simulink model "AutonomousModel_V1"  (R2020b)
settings: Solver=ode23t  StartTime=0.0  StopTime=180.1  FixedStep=0.05  RelTol=1e-3  EnableMultiTasking=on
model workspace (MAT data in the model file):
  occGrid = robotics.BinaryOccupancyGrid
  occGrid.Grid = [1 1 1 1 1 1 1 1 1 1 1 1 ... (4194304 elements, 2048x2048)]
  occGrid.LayerName = "binaryLayer"
  occGrid.Index = matlabshared.autonomous.internal.CircularBufferIndex
  occGrid.Index.Head = [1 1]
  occGrid.Index.Size = [2048 2048]
  occGrid.Index.NewRegions = [0 0 0 0]
  occGrid.Index.DropEntireMap = 0
  occGrid.Index.DropTwoRegions = [0 0]
  occGrid.Buffer = matlabshared.autonomous.internal.CircularBuffer
  occGrid.Buffer.ConstVal = 0
  occGrid.Buffer.DataType = 'logical'
  occGrid.Buffer.Index = matlabshared.autonomous.internal.CircularBufferIndex
  occGrid.Buffer.Index.Head = [1 1]
  occGrid.Buffer.Index.Size = [2048 2048]
  occGrid.Buffer.Index.NewRegions = [0 0 0 0]
  occGrid.Buffer.Index.DropEntireMap = 0
  occGrid.Buffer.Index.DropTwoRegions = [0 0]
  occGrid.Buffer.Buffer = [1 1 1 1 1 1 1 1 1 1 1 1 ... (4194304 elements, 2048x2048)]
  occGrid.DefaultValueInternal = 0
  occGrid.HasParent = 0
  occGrid.Resolution = 409.6
  occGrid.GridSize = [2048 2048]
  occGrid.GridOriginInLocal = [0 0]
  occGrid.LocalOriginInWorld = [0 0]
  occGrid.Width = 5
  occGrid.Height = 5
  occGrid.LocalOriginInWorldInternal = [0 0]
undefined symbols (not defined in the file): cellLevel, cellPose, cellTypeArray, FloorSurface, isoPoses, platformPoses, PlowSurface, Ref, RobotSurface, WallSurface, X, Y, Z
libraries: sm_lib x286, nesl_utility x157, simulink x72, simulink_extras x2, pid_lib x2
(part 1 of 14)
settings Model: DataTypeOverride=Off  MinMaxOverflowLogging=ForceOff  EnablePacing=on  PacingRate=1000  ExtModeTrigDuration=25  OrderedModelArguments=off  Creator=scastro  LastModifiedBy=wanga
settings SolverCC: AlgebraicLoopSolver=LineSearch
settings DataIOCC: LimitDataPoints=on  SignalLogging=off  ReturnWorkspaceOutputs=off
settings OptimizationCC: DefaultParameterBehavior=Inlined  PassReuseOutputArgsAs=Individual arguments  MaxStackSize=64  EfficientTunableParamExpr=on
settings DebuggingCC: ReadBeforeWriteMsg=DisableAll  WriteAfterWriteMsg=DisableAll  WriteAfterReadMsg=DisableAll  MultiTaskDSMMsg=none  ParameterPrecisionLossMsg=none  ParameterTunabilityLossMsg=error  UnconnectedLineMsg=none  AllowSymbolicDim=off  SFUnexpectedBacktrackingDiag=warning  SFNoUnconditionalDefaultTransitionDiag=warning  SFExecutionAtInitializationDiag=none  ArithmeticOperatorsInVariantConditions=warning
settings HardwareCC: ProdBitPerPointer=32  ProdBitPerSizeT=32  ProdBitPerPtrDiffT=32  ProdLargestAtomicInteger=Long  ProdLargestAtomicFloat=Double  ProdWordSize=32  ProdHWDeviceType=ARM Compatible->ARM Cortex
settings ModelReferenceCC: UpdateModelReferenceTargets=IfOutOfDate
settings SFSimCC: SFSimEcho=off  SimUseLocalCustomCode=off  MATLABDynamicMemAlloc=off  CustomCodeUndefinedFunction=UseInterfaceOnly
settings RTWCC: Description=Embedded Coder  SystemTargetFile=ert.tlc  TemplateMakefile=ert_default_tmf  GenerateReport=on  RTWUseLocalCustomCode=off  Toolchain=GNU Tools for ARM Embedded Processors  IncludeHyperlinkInReport=on  LaunchReport=on  GenerateTraceInfo=on  GenerateTraceReport=on  GenerateTraceReportSl=on  GenerateTraceReportSf=on  GenerateTraceReportEml=on
settings CodeAppCC: ForceParamTrailComments=on  IgnoreCustomStorageClasses=off  OperatorAnnotations=on  SimulinkDataObjDesc=on  SFDataObjDesc=on  InsertBlockDesc=on
settings ERTTargetCC: ExtModeStaticAllocSize=2048  ERTCustomFileTemplate=example_file_process.tlc
settings ConfigComp: CovMetricSettings=dw  CovSaveCumulativeToWorkspaceVar=on  CovSaveSingleToWorkspaceVar=on  CovExternalEMLEnable=off  CovSFcnEnable=off
settings SimscapeCC: SimscapeNominalValues="[{\"value\":\"10\",\"unit\":\"V\"},{\"value\":\"1\",\"unit\":\"A\"},{\"value\":\"10\",\"unit\":\"N*m\"},{\"value\":\"10\",\"unit\":\"bar\"},{\"value\":\"100\",\"unit\":\"kJ/kg\"},{\"value\":\"1\",\"unit\":\"kW\"},{\"value\":\"300\",\"unit\":\"K\"},{\"value\":\"100\",\"unit\":\"cm^3/s\"},{\"value\":\"1\",\"unit\":\"kN\"},{\"value\":\"1\",\"unit\":\"g/cm^3\"},{\"value\":\"1\",\"unit\":\"l\"},{\"value\":\"1\",\"unit\":\"cm^2\"},{\"value\":\"60\",\"unit\":\"Hz\"}]"  SimscapeLogOpenViewer=on  SimscapeLogDataHistory=10000
settings ConfigurationSet: Description=SimMechanics 2G
settings DiagnosticsConfigSet: SimMechanicsRigidlyBoundBlock=none
settings ExplorerConfigSet: InternalSimMechanicsExplorerSettings="<ExplorerConfiguration><canonicalview>default</canonicalview><AnimationSetting><BasePlaybackSpeed>1.0</BasePlaybackSpeed><PlaybackSpeedFactor>1.0</PlaybackSpeedFactor></AnimationSetting><TilePanel><TileInfo><Tiles Columns=\"2\" Count=\"3\" Rows=\"2\"><Column Weight=\"0.5\"/><Column Weight=\"0.5\"/><Row Weight=\"0.6225\"/><Row Weight=\"0.3775\"/><Tile Height=\"1\" Width=\"2\" X=\"0\" Y=\"0\"/><Tile Height=\"1\" Width=\"1\" X=\"0\" Y=\"1\"/><Tile Height=\"1\" Width=\"1\" X=\"1\" Y=\"1\"/></Tiles></TileInfo><SceneInfo><SceneViewer><BGColor><R>0.60000002384185791</R><G>0.60000002384185791</G><B>0.60000002384185791</B></BGColor><Camera><DoPerspective>on</DoPerspective><Position><X>-2.5</X><Y>0</Y><Z>0.469999999999999973</Z></Position><Center><X>-1.56030737921409157</X><Y>0</Y><Z>0.12797985667433126</Z></Center><Up><X>0.342020143325668713</X><Y>0</Y><Z>0.939692620785908428</Z></Up><ViewLimDist>1</ViewLimDist><YLim>0.466307658154998583</YLim><XLim>1.13267634384101279</XLim></Camera></SceneViewer><SceneViewer><BGColor><R>0.60000002384185791</R><G>0.60000002384185791</G><B>0.60000002384185791</B></BGColor><Camera><DoPerspective>off</DoPerspective><Position><X>3.5332314785771386</X><Y>-3.3947402734829315</Y><Z>3.53231830664862745</Z></Position><Center><X>0.446325858412655041</X><Y>-0.728979182990680097</Y><Z>0.58226398573312621</Z></Center><Up><X>-0.344859316417843731</X><Y>0.487999196814355329</Y><Z>0.801828432888458731</Z></Up><ViewLimDist>1</ViewLimDist><YLim>1.33865160703358899</YLim><XLim>2.67730321406717797</XLim></Camera></SceneViewer><SceneViewer><BGColor><R>0.60000002384185791</R><G>0.60000002384185791</G><B>0.60000002384185791</B></BGColor><Camera><DoPerspective>off</DoPerspective><Position><X>-0.106931959652509123</X><Y>-0.225697807623169988</Y><Z>4.9870492424192383</Z></Position><Center><X>-0.106931959652509123</X><Y>-0.225697807623169988</Y><Z>0.219820364094227116</Z></Center><Up><X>0</X><Y>1</Y><Z>-0</Z></Up><ViewLimDist>1</ViewLimDist><YLim>1.8966863569500001</YLim><XLim>3.79337271390000019</XLim></Camera></SceneViewer></SceneInfo></TilePanel><MechEditorPanel><Cameras><Camera><Id>Camera1</Id><Value><Name>RobotView</Name><NativeCamera><PositionTrackingFeature>BEST_Robotics_2020_Game_Double_Click.BEST_2020_Robot.Body.RobotCamera.F</PositionTrackingFeature><CenterTrackingFeature>BEST_Robotics_2020_Game_Double_Click.BEST_2020_Robot.Body.RobotCamera.F</CenterTrackingFeature><UpVectorTrackingFeature>BEST_Robotics_2020_Game_Double_Click.BEST_2020_Robot.Body.RobotCamera.F</UpVectorTrackingFeature><CenterTrackingOrigin>off</CenterTrackingOrigin><CenterTrackingDirection>+X</CenterTrackingDirection><UpVectorTrackingDirection>+Z</UpVectorTrackingDirection></NativeCamera></Value></Camera></Cameras><GfxPanelCameraMap><MapElement CameraMLId=\"Camera1\" GfxPanelIndex=\"0\"/></GfxPanelCameraMap><VideoCreator><PlaybackSpeedRatio>1.0</PlaybackSpeedRatio><FrameRate>16</FrameRate><VideoFormat>Motion JPEG AVI</VideoFormat><FrameSize>auto</FrameSize></VideoCreator></MechEditorPanel></ExplorerConfiguration>"

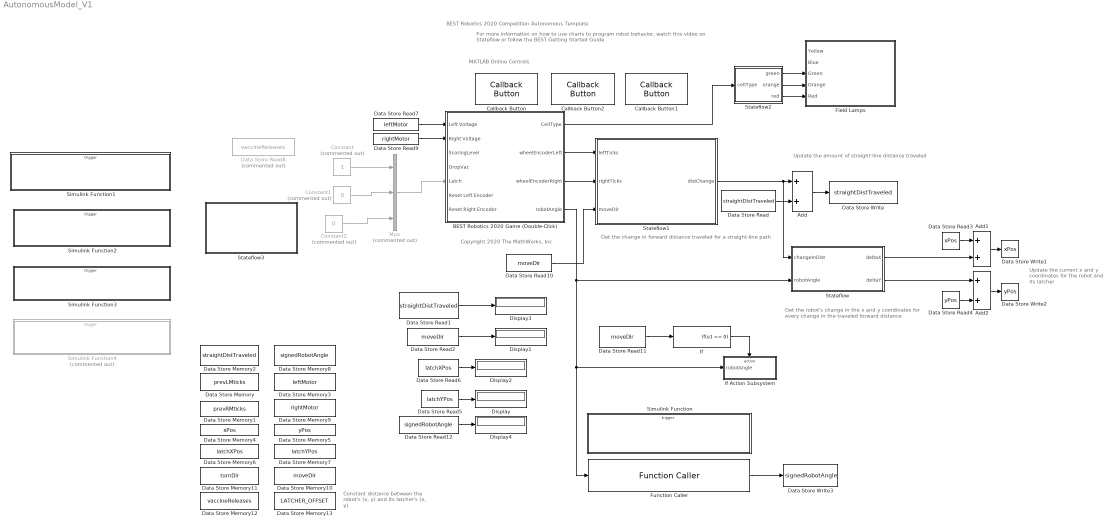
== system AutonomousModel_V1 ==
  note: Update the current x and y coordinates for the robot and its latcher
  note: Get the robot's change in the x and y coordinates for
      | every change in the traveled forward distance
  note: Update the amount of straight-line distance traveled
  note: Get the change in forward distance traveled for a straight-line path
  note: MATLAB Online Controls
  note: For more information on how to use charts to program robot behavior,
      | watch this video on Stateflow or follow the BEST Getting Started Guide
  note: BEST Robotics 2020 Competition Autonomous Template
  note: Copyright 2020 The MathWorks, Inc
  note: Constant distance between the robot's (x, y) and
      | its latcher's (x, y)
  Add : Sum
  Add1 : Sum
  Add2 : Sum
  BEST Robotics 2020 Game (Double-Click) : Subsystem  mask(RP BEST Robotics 2020 Challenge){gameTime=180, field=Practice 3, rvis=off, sensor=off, autoField=on, wheelBase=0.5, wheelRadius=0.1, robotColor=[0.5 0 0], wheelThickness=0.025, chassisThickness=0.05, wheelMass=1, chassisMass=1.5}
      mask prompts: gameTime "Game Time (s)"; field "Field Layout"; rvis "Show cell type after run (Runs slower)"; sensor "Activate Gripper Sensor (Not allowed during competition)"; autoField "Autonomous Configuration"; wheelBase "Distance between wheels [m]"; wheelRadius "Wheel radius [m]"; robotColor "Color [R G B]"; wheelThickness "Wheel Thickness [m]"; chassisThickness "Chassis Thickness [m]"; wheelMass "Wheel Mass [kg]"; chassisMass "Chassis Mass [kg]"
      mask help:
      | This block contains a virtual game for the BEST Robotics 2020 competition. Please refere to the instructions provided by competition organizers for more information on game rules.
      |
      | Inputs:
      | Motor Voltages (Torque) [-127 to 127]
      | LatchCell (Pickup Cell) [0 or 1]
      | ScoringLevel (Floor or Platform) [0 or 1]
      | DropVac (Release vaccine) [0 or 1] Array of 3
      |
      | Outputs:
      | Cell Type (Uninfected, Immune, Infected) [0 ,1 or 2]
      | Sensors (See inside block for sensor properties and outputs)
      |
      | For MATLAB and Simulink related questions please email: roboticsarena@mathworks.com
      mask init:
      | autochoice=get_param(gcb,'autoField');
      | choice=get_param(gcb,'field');
      | time=get_param(gcb,'gameTime');
      | set_param(gcs,'StopTime',num2str(str2num(time)+0.1));
      | 
      | if strcmp(choice,'Practice 1')
      |   BEST2020GameConfig1 
      | elseif strcmp(choice,'Practice 2')
      |   BEST2020GameConfig2 
      | elseif strcmp(choice,'Practice 3')
      |   BEST2020GameConfig3 
      | elseif strcmp(choice,'Random')
      |   BEST2020GameConfigRand
      | elseif strcmp(autochoice,"on")
      |    if strcmp(choice,'Competition 1 (Provided during competition)')
      |      BEST2020GameConfigAuto1
      |    elseif strcmp(choice,'Competition 2 (Provided during competition)')
      |      BEST2020GameConfigAuto2
      |    elseif strcmp(choice,'Competition 3 (Provided during competition)')
      |      BEST2020GameConfigAuto3
      |    elseif strcmp(choice,'Competition 4 (Provided during competition)')
      |      BEST2020GameConfigAuto4
      |    elseif strcmp(choice,'Competition 5 (Provided during competition)')
      |      BEST2020GameConfigAuto5
      |    elseif strcmp(choice,'Competition 6 (Provided during competition)')
      |      BEST2020GameConfigAuto6
      |    elseif strcmp(choice,'Competition 7 (Provided during competition)')
      |      BEST2020GameConfigAuto7
      |    elseif strcmp(choice,'Competition 8 (Provided during competition)')
      |      BEST2020GameConfigAuto8
      |    else
      |      BEST2020GameConfigAuto1
      |    end
      | elseif strcmp(choice,'Competition 1 (Provided during competition)')
      |   BEST2020GameConfigComp1
      | elseif strcmp(choice,'Competition 2 (Provided during competition)')
      |   BEST2020GameConfigComp2
      | elseif strcmp(choice,'Competition 3 (Provided during competition)')
      |   BEST2020GameConfigComp3
      | elseif strcmp(choice,'Competition 4 (Provided during competition)')
      |   BEST2020GameConfigComp4
      | elseif strcmp(choice,'Competition 5 (Provided during competition)')
      |   BEST2020GameConfigComp5
      | elseif strcmp(choice,'Competition 6 (Provided during competition)')
      |   BEST2020GameConfigComp6
      | elseif strcmp(choice,'Competition 7 (Provided during competition)')
      |   BEST2020GameConfigComp7
      | elseif strcmp(choice,'Competition 8 (Provided during competition)')
      |   BEST2020GameConfigComp8
      | else
      |   BEST2020GameConfig1 
      | end
      mask TypeOptions field: Practice 1 | Practice 2 | Practice 3 | Random | Competition 1 (Provided during competition) | Competition 2 (Provided during competition) | Competition 3 (Provided during competition) | Competition 4 (Provided during competition) | Competition 5 (Provided during competition) | Competition 6 (Provided during competition) | Competition 7 (Provided during competition) | Competition 8 (Provided during competition)
      mask Callback rvis:
      | visual=get_param(gcb,'rvis');
      | for i=1:21
      |     if strcmp(visual,'off')
      |         set_param([gcb '/Cells/Object' num2str(i) '/EndVisuals'],'Commented','on');
      |     else
      |         set_param([gcb '/Cells/Object' num2str(i) '/EndVisuals'],'Commented','off');
      |     end
      | end
      mask TypeOptions wheelThickness: BEST 2020 Robot/wheelThickness
      mask TypeOptions chassisThickness: BEST 2020 Robot/chassisThickness
      mask TypeOptions wheelMass: BEST 2020 Robot/wheelMass
      mask TypeOptions chassisMass: BEST 2020 Robot/chassisMass
      mask DialogControl Container8 Prompt: Game Settings
      mask DialogControl Container4 Prompt: Robot settings
      mask Display:
      | image('BEST2020Environment.png')
      | port_label('input',1,'LeftMotor')
      | port_label('input',2,'RightMotor')
      | port_label('input',3,'LatchCell')
      | port_label('input',4,'ScoringLevel')
      | port_label('input',5,'DropVac')
      | port_label('output',1,'CellType')
      | port_label('output',2,'LeftEncoder')
      | port_label('output',3,'RightEncoder')
      | port_label('output',4,'RobotAngle')
  Callback Button : CallbackButton  ButtonText=Create Simulation Video (FPV)
      settings: ClickFcn=|
      | %% Simulate Model and Create Video
      | model=gcs;
      | disp(['Simulating Model: ' model '...'])
      | w=waitbar(0,['Simulating Model: ' model '...']);
      | set_param(model, 'EnablePacing', 'off');
      | sim(model);
      | set_param(model, 'EnablePacing', 'on');
      | disp('Creating Simulation Video...')
      | waitbar(0.5,w,'Creating Simulation Video...')
      | smwritevideo(model,model,'FrameRate',16,'FrameSize',[1280 720],'Tile',1)
      | disp('Animation window will close when completed')
      | waitbar(1,w,'Animation window will close when completed')
      | pause(5)
      | close(w)
  Callback Button1 : CallbackButton  ButtonText=Re-play Simulation Video
      settings: ClickFcn=|
      | %% Playback Simulation Video
      | disp('Replaying Simulation Video...')
      | videoReader = VideoReader([gcs '.avi']);
      | videoPlayer = vision.VideoPlayer('Position',[100 100 1280 720]);
      | 
      | % Play video. Every call to the step method reads another frame.
      | 
      | while hasFrame(videoReader)
      |    frame = readFrame(videoReader);
      |    step(videoPlayer,frame);
      |    pause(1/16);
      | end
      | disp('Done replaying simulation video')
  Callback Button2 : CallbackButton  ButtonText=Create Simulation Video (Top View)
      settings: ClickFcn=|
      | %% Simulate Model and Create Video
      | model=gcs;
      | disp(['Simulating Model: ' model '...'])
      | w=waitbar(0,['Simulating Model: ' model '...']);
      | set_param(model, 'EnablePacing', 'off');
      | sim(model);
      | set_param(model, 'EnablePacing', 'on');
      | disp('Creating Simulation Video...')
      | waitbar(0.5,w,'Creating Simulation Video...')
      | smwritevideo(model,model,'FrameRate',16,'FrameSize',[1280 720],'Tile',3)
      | disp('Animation window will close when completed')
      | waitbar(1,w,'Animation window will close when completed')
      | pause(5)
      | close(w)
  Constant : Constant  Commented=on
  Constant1 : Constant  Commented=on  Value=0
  Constant2 : Constant  Commented=on  Value=0
  Data Store Memory1 : DataStoreMemory  DataStoreName=prevRMticks  ReadBeforeWriteMsg=warning  WriteAfterWriteMsg=warning  WriteAfterReadMsg=warning  ShowAdditionalParam=off  OutDataTypeStr=double  Dimensions=1
  Data Store Memory10 : DataStoreMemory  DataStoreName=moveDir  ReadBeforeWriteMsg=warning  WriteAfterWriteMsg=warning  WriteAfterReadMsg=warning  ShowAdditionalParam=off  OutDataTypeStr=double  Dimensions=1
  Data Store Memory11 : DataStoreMemory  DataStoreName=turnDir  ReadBeforeWriteMsg=warning  WriteAfterWriteMsg=warning  WriteAfterReadMsg=warning  ShowAdditionalParam=off  OutDataTypeStr=double  Dimensions=1
  Data Store Memory12 : DataStoreMemory  DataStoreName=vaccineReleases  ReadBeforeWriteMsg=warning  WriteAfterWriteMsg=warning  WriteAfterReadMsg=warning  InitialValue=[0 0 0]  VectorParams1D=off  ShowAdditionalParam=off  OutDataTypeStr=double  Dimensions=[1 3]
      settings: LockScale=on
  Data Store Memory13 : DataStoreMemory  DataStoreName=LATCHER_OFFSET  ReadBeforeWriteMsg=warning  WriteAfterWriteMsg=warning  WriteAfterReadMsg=warning  InitialValue=0.3812987013  ShowAdditionalParam=off  OutDataTypeStr=double  Dimensions=1
  Data Store Memory2 : DataStoreMemory  DataStoreName=straightDistTraveled  ReadBeforeWriteMsg=warning  WriteAfterWriteMsg=warning  WriteAfterReadMsg=warning  ShowAdditionalParam=off
  Data Store Memory3 : DataStoreMemory  DataStoreName=leftMotor  ReadBeforeWriteMsg=warning  WriteAfterWriteMsg=warning  WriteAfterReadMsg=warning  ShowAdditionalParam=off  OutDataTypeStr=double  Dimensions=1
  Data Store Memory4 : DataStoreMemory  DataStoreName=xPos  ReadBeforeWriteMsg=warning  WriteAfterWriteMsg=warning  WriteAfterReadMsg=warning  InitialValue=-0.4071428571  ShowAdditionalParam=off  OutDataTypeStr=double  Dimensions=1
  Data Store Memory5 : DataStoreMemory  DataStoreName=yPos  ReadBeforeWriteMsg=warning  WriteAfterWriteMsg=warning  WriteAfterReadMsg=warning  InitialValue=1.6  ShowAdditionalParam=off  OutDataTypeStr=double  Dimensions=1
  Data Store Memory6 : DataStoreMemory  DataStoreName=latchXPos  ReadBeforeWriteMsg=warning  WriteAfterWriteMsg=warning  WriteAfterReadMsg=warning  InitialValue=-0.4071428571  ShowAdditionalParam=off  OutDataTypeStr=double  Dimensions=1
  Data Store Memory7 : DataStoreMemory  DataStoreName=latchYPos  ReadBeforeWriteMsg=warning  WriteAfterWriteMsg=warning  WriteAfterReadMsg=warning  InitialValue=1.6  ShowAdditionalParam=off  OutDataTypeStr=double  Dimensions=1
  Data Store Memory8 : DataStoreMemory  DataStoreName=signedRobotAngle  ReadBeforeWriteMsg=warning  WriteAfterWriteMsg=warning  WriteAfterReadMsg=warning  ShowAdditionalParam=off  Dimensions=1
  Data Store Memory9 : DataStoreMemory  DataStoreName=rightMotor  ReadBeforeWriteMsg=warning  WriteAfterWriteMsg=warning  WriteAfterReadMsg=warning  ShowAdditionalParam=off  OutDataTypeStr=double  Dimensions=1
  Data Store Read : DataStoreRead  DataStoreName=straightDistTraveled
  Data Store Read1 : DataStoreRead  DataStoreName=straightDistTraveled
  Data Store Read10 : DataStoreRead  DataStoreName=moveDir
  Data Store Read11 : DataStoreRead  DataStoreName=moveDir
  Data Store Read12 : DataStoreRead  DataStoreName=signedRobotAngle
  Data Store Read2 : DataStoreRead  DataStoreName=moveDir
  Data Store Read3 : DataStoreRead  DataStoreName=xPos
  Data Store Read4 : DataStoreRead  DataStoreName=yPos
  Data Store Read5 : DataStoreRead  DataStoreName=latchYPos
  Data Store Read6 : DataStoreRead  DataStoreName=latchXPos
  Data Store Read7 : DataStoreRead  DataStoreName=leftMotor
  Data Store Read8 : DataStoreRead  Commented=on  DataStoreName=vaccineReleases
  Data Store Read9 : DataStoreRead  DataStoreName=rightMotor
  Data Store Write : DataStoreWrite  DataStoreName=straightDistTraveled
  Data Store Write1 : DataStoreWrite  DataStoreName=xPos
  Data Store Write2 : DataStoreWrite  DataStoreName=yPos
  Data Store Write3 : DataStoreWrite  DataStoreName=signedRobotAngle
  Data Store Memory : DataStoreMemory  DataStoreName=prevLMticks  ReadBeforeWriteMsg=warning  WriteAfterWriteMsg=warning  WriteAfterReadMsg=warning  ShowAdditionalParam=off  OutDataTypeStr=double  Dimensions=1
  Display{,1..4} (5 alike) : Display
  Field Lamps : Subsystem
      mask Display:
      | image('lamps.PNG')
      | port_label('input',1,'Yellow')
      | port_label('input',2,'Blue')
      | port_label('input',3,'Green')
      | port_label('input',4,'Orange')
      | port_label('input',5,'Red')
  Function Caller : FunctionCaller  FunctionPrototype=signedRobotAngle = getSignedRobotAngle(robotAngle)  InputArgumentSpecifications=<Enter example>  OutputArgumentSpecifications=<Enter example>
  If : If  IfExpression=u1 == 0  ShowElse=off
  If Action Subsystem : Subsystem  TreatAsAtomicUnit=on
  Mux : Mux  Commented=on  Inputs=3
  Simulink Function : Subsystem  TreatAsAtomicUnit=on
  Simulink Function1 : Subsystem  TreatAsAtomicUnit=on
  Simulink Function2 : Subsystem  TreatAsAtomicUnit=on
  Simulink Function3 : Subsystem  TreatAsAtomicUnit=on
  Simulink Function4 : Subsystem  Commented=on  TreatAsAtomicUnit=on
  Stateflow : Stateflow chart  TreatAsAtomicUnit=on
  Stateflow1 : Stateflow chart  TreatAsAtomicUnit=on
  Stateflow2 : Stateflow chart  TreatAsAtomicUnit=on
  Stateflow3 : Stateflow chart  TreatAsAtomicUnit=on
  wires:
  BEST Robotics 2020 Game (Double-Click)/3(wheelEncoderRight) -> Stateflow1/2(rightTicks)
  BEST Robotics 2020 Game (Double-Click)/2(wheelEncoderLeft) -> Stateflow1/1(leftTicks)
  BEST Robotics 2020 Game (Double-Click)/1(CellType) -> Stateflow2/1(cellType)
  Stateflow2/1(green) -> Field Lamps/3(Green)
  Stateflow2/3(red) -> Field Lamps/5(Red)
  Stateflow2/2(orange) -> Field Lamps/4(Orange)
  Stateflow1/1(distChange) -> Stateflow/1(changeInDist), Add/1
  Data Store Read/1 -> Add/2
  Add/1 -> Data Store Write/1
  Data Store Read1/1 -> Display3/1
  Stateflow/1(deltaX) -> Add1/2
  Add1/1 -> Data Store Write1/1
  Stateflow/2(deltaY) -> Add2/1
  Add2/1 -> Data Store Write2/1
  Data Store Read3/1 -> Add1/1
  Data Store Read4/1 -> Add2/2
  Function Caller/1 -> Data Store Write3/1
  If/1 -> If Action Subsystem/Action
  BEST Robotics 2020 Game (Double-Click)/4(robotAngle) -> Stateflow/2(robotAngle), Function Caller/1, If Action Subsystem/1(robotAngle)
  Data Store Read7/1 -> BEST Robotics 2020 Game (Double-Click)/1(Left Voltage)
  Data Store Read9/1 -> BEST Robotics 2020 Game (Double-Click)/2(Right Voltage)
  Data Store Read10/1 -> Stateflow1/3(moveDir)
  Data Store Read11/1 -> If/1
  Data Store Read2/1 -> Display1/1
  Data Store Read5/1 -> Display/1
  Data Store Read6/1 -> Display2/1
  Data Store Read12/1 -> Display4/1
  Mux/1 -> BEST Robotics 2020 Game (Double-Click)/5(Latch)
  Constant/1 -> Mux/1
  Constant1/1 -> Mux/2
  Constant2/1 -> Mux/3

== system AutonomousModel_V1/BEST Robotics 2020 Game (Double-Click) ==
  note: DO NOT CHANGE THIS MODEL!
  Left Voltage : Inport
  Right Voltage : Inport  Port=2
  ScoringLevel : Inport  Port=3
  DropVac : Inport  Port=4
  Latch : Inport  Port=5
  Reset Left Encoder : Inport  Port=6
  Reset Right Encoder : Inport  Port=7
  Arena : Subsystem  mask(RP Grid Arena){length=7, width=7}
      mask prompts: length "Arena length [m]"; width "Arena width [m]"
      mask help: This block is an arena for robots to operate within. This arena implements contact between one robot and the walls and also introduces a floor grid for better visualization. Connect to other robots within the library using the corresponding "Robot" and "Ref" ports.
      mask DialogControl Container5 Prompt: Arena dimensions
      mask Display:
      | image('BEST2020Arena.png')
      | port_label('Lconn',1,'RP-Bus')
  BEST 2020 Robot : Subsystem  mask(RP Contact Tank Robot){robotId=1, wheelRadius=wheelRadius, wheelBase=wheelBase, wheelThickness=wheelThickness, chassisThickness=chassisThickness, startPose=[-2 0], choice=off, sensorTs=0.05, wheelMass=wheelMass, chassisMass=chassisMass, maxWheelTorque=2, wheelColor=[0.25 0.25 0.25], chassisColor=robotColor}
      mask prompts: robotId "Robot ID"; wheelRadius "Wheel Radius [m]"; wheelBase "Wheelbase [m]"; wheelThickness "Wheel Thickness [m]"; chassisThickness "Chassis Thickness [m]"; startPose "Start Position [m]"; choice "Reverse Start Position"; sensorTs "Sensor sample time [s]"; wheelMass "Wheel Mass [kg]"; chassisMass "Chassis Mass [kg]"; maxWheelTorque "Maximum wheel torque [N*m]"; wheelColor "Wheel Color"; chassisColor "Chassis Color"
      mask help:
      | This robot implements contact between the robot wheels and the floor of an arena. The stck-slip friction implemented using contact force libraries makes the robot behavior more realistic. The inputs to the robot are now motor torque, which is set using the Robotics Playground Motor blocks. The motor mappings are as follows:
      |
      | Motor 1 -> Left wheel motor torque
      | Motor 2 -> Right wheel motor torque
      mask DialogControl KinContainer Prompt: Kinematics
      mask DialogControl DynamicsContainer Prompt: Dynamics
      mask DialogControl AppearanceContainer Prompt: Appearance
      mask Display:
      | image('BEST2020Robot.png')
      | port_label('Rconn',1,'RP-Bus')
  Cells : Subsystem
      mask Display: image('BEST2020Cells.png')
  Compass Sensor : Subsystem  mask(RP Compass Sensor){sensorTs=0.1}
      mask prompts: sensorTs "Sensor sample time [s]"
      mask help: This sensor outputs the rotation in degrees as measured from the robot center relative to the world coordinate frame.
      mask Help: web('compass_sensor.htm')
      mask DialogControl senCont Prompt: Sensor Characteristics
      mask Display:
      | color('white');
      | plot([100,100,100,100]*1,[100,100,100,100]*1);
      | plot([100,100,100,100]*0,[100,100,100,100]*0);
      | image('Compass.png','center')
      | color('blue');
  Game Control : Subsystem
  Left Encoder : Subsystem  mask(RP Motor Encoder){rstChoice=No reset, ticks=180, detectDir=off, sensorTs=0.1}
      mask prompts: rstChoice "Reset option"; ticks "Ticks per rotation"; detectDir "Detect direction of rotation"; sensorTs "Sensor sample time [s]"
      mask help:
      | This block outputs the rotation in tick counts of an encoder conneted to the respective robot motor. You can set different sensor parameters from the mask or use the default settings.
      |
      | The most common use of motor encoders is to derive the position of an object. Start by converting the tick counts to revolutions of the motor shaft. You can later relate the revolutions of the motor shaft to more valuable robot information such as traveled distance by using robot dimensions like the wheel size.
      mask Help: web('encoder_sensor.htm')
      mask TypeOptions rstChoice: No reset | Reset by external signal
      mask DialogControl ParameterGroupVar Prompt: Settings
      mask Display:
      | color('white');
      | plot([100,100,100,100]*1,[100,100,100,100]*1);
      | plot([100,100,100,100]*0,[100,100,100,100]*0);
      | image('encoder.jpg','center')
  Right Encoder : Subsystem  mask(RP Motor Encoder){rstChoice=No reset, ticks=180, detectDir=off, sensorTs=0.1}
      mask prompts: rstChoice "Reset option"; ticks "Ticks per rotation"; detectDir "Detect direction of rotation"; sensorTs "Sensor sample time [s]"
      mask help:
      | This block outputs the rotation in tick counts of an encoder conneted to the respective robot motor. You can set different sensor parameters from the mask or use the default settings.
      |
      | The most common use of motor encoders is to derive the position of an object. Start by converting the tick counts to revolutions of the motor shaft. You can later relate the revolutions of the motor shaft to more valuable robot information such as traveled distance by using robot dimensions like the wheel size.
      mask Help: web('encoder_sensor.htm')
      mask TypeOptions rstChoice: No reset | Reset by external signal
      mask DialogControl ParameterGroupVar Prompt: Settings
      mask Display:
      | color('white');
      | plot([100,100,100,100]*1,[100,100,100,100]*1);
      | plot([100,100,100,100]*0,[100,100,100,100]*0);
      | image('encoder.jpg','center')
  Vaccines : Subsystem
      mask Display: image('BEST2020Vaccines.png')
  CellType : Outport
  wheelEncoderLeft : Outport  Port=2
  wheelEncoderRight : Outport  Port=3
  robotAngle : Outport  Port=4
  wires:
  Right Voltage/1 -> BEST 2020 Robot/2(In2)
  Left Voltage/1 -> BEST 2020 Robot/1(In1)
  Latch/1 -> Cells/1(Latch)
  Cells/1(CellType) -> CellType/1
  Right Encoder/1(Out1) -> wheelEncoderRight/1
  Left Encoder/1(Out1) -> wheelEncoderLeft/1
  BEST 2020 Robot/1(leftMotorW) -> Left Encoder/1(In1)
  BEST 2020 Robot/2(rightMotorW) -> Right Encoder/1(In1)
  BEST 2020 Robot/3(angle) -> Compass Sensor/1(angle)
  Compass Sensor/1(Distance) -> robotAngle/1
  DropVac/1 -> Vaccines/2(Drop)
  ScoringLevel/1 -> Vaccines/1("ScoreLevel "), Cells/2(ScoringLevel)
  Reset Left Encoder/1 -> Left Encoder/2(Input)
  Reset Right Encoder/1 -> Right Encoder/2(Input)
  connections:
  Vaccines/LConn1 -- Arena/LConn1 -- BEST 2020 Robot/RConn1 -- Cells/LConn1

== system AutonomousModel_V1/Field Lamps ==
  note: DO NOT EDIT
  note: Inputs should be 0 or 1
  Yellow : Inport
  Blue : Inport  Port=2
  Green : Inport  Port=3
  Orange : Inport  Port=4
  Red : Inport  Port=5
  tag scope: blueLamp=global, greenLamp=global, orangeLamp=global, redLamp=global, yellowLamp=global
  wires:
  Yellow/1 -> [yellowLamp]
  Blue/1 -> [blueLamp]
  Orange/1 -> [orangeLamp]
  Red/1 -> [redLamp]
  Green/1 -> [greenLamp]

== system AutonomousModel_V1/If Action Subsystem ==
  robotAngle : Inport
  Action Port : ActionPort  ActionPortLabel=if(u1 == 0)
  Add : Sum
  Add1 : Sum
  Cos : Trigonometry  Operator=cos
  Data Store Read1 : DataStoreRead  DataStoreName=LATCHER_OFFSET
  Data Store Read12 : DataStoreRead  DataStoreName=xPos
  Data Store Read13 : DataStoreRead  DataStoreName=yPos
  Data Store Read8 : DataStoreRead  DataStoreName=turnDir
  Data Store Write4 : DataStoreWrite  DataStoreName=latchXPos
  Data Store Write5 : DataStoreWrite  DataStoreName=latchYPos
  Degrees to Radians : simulink_extras/Transformations/Degrees to Radians
  Product : Product  RndMeth=Zero
  Product1 : Product  RndMeth=Zero
  Product2 : Product  RndMeth=Zero
  Sin : Trigonometry
  wires:
  robotAngle/1 -> Product/1
  Degrees to Radians/1 -> Sin/1, Cos/1
  Cos/1 -> Product1/1
  Data Store Read1/1 -> Product2/1, Product1/2
  Sin/1 -> Product2/2
  Add/1 -> Data Store Write4/1
  Product1/1 -> Add/2
  Data Store Read12/1 -> Add/1
  Product2/1 -> Add1/1
  Data Store Read13/1 -> Add1/2
  Add1/1 -> Data Store Write5/1
  Data Store Read8/1 -> Product/2
  Product/1 -> Degrees to Radians/1

== system AutonomousModel_V1/Simulink Function ==
  getSignedRobotAngle : TriggerPort  TriggerType=function-call  IsSimulinkFunction=on  FunctionName=getSignedRobotAngle  FunctionVisibility=scoped  VariantControl=(inherit)
  Data Store Read8 : DataStoreRead  DataStoreName=yPos
  Data Store Read9 : DataStoreRead  DataStoreName=latchYPos
  Product : Product  RndMeth=Zero
  Sign : Signum
  Subtract1 : Sum  Inputs=+-
  robotAngle : ArgIn  DisableCoverage=on  ArgumentName=robotAngle
  signedRobotAngle : ArgOut  DisableCoverage=on  ArgumentName=signedRobotAngle
  wires:
  Data Store Read9/1 -> Subtract1/1
  Data Store Read8/1 -> Subtract1/2
  Subtract1/1 -> Sign/1
  robotAngle/1 -> Product/2
  Sign/1 -> Product/1
  Product/1 -> signedRobotAngle/1

== system AutonomousModel_V1/Simulink Function1 ==
  note: PID_SETTLE_TIME is measured in n*0.1 seconds,
      | meaning a value of 5 for this would mean a
      | requirement for the PID to turn the robot should
      | settle for 0.5 seconds before stopping
  hasMovedDist : TriggerPort  TriggerType=function-call  IsSimulinkFunction=on  FunctionName=hasMovedDist  FunctionVisibility=scoped  VariantControl=(inherit)
  Abs1 : Abs
  Data Store Memory : DataStoreMemory  DataStoreName=PID_DIST_TOLERANCE  ReadBeforeWriteMsg=warning  WriteAfterWriteMsg=warning  WriteAfterReadMsg=warning  InitialValue=0.003  ShowAdditionalParam=off
  Data Store Memory1 : DataStoreMemory  DataStoreName=PID_SETTLE_TIME  ReadBeforeWriteMsg=warning  WriteAfterWriteMsg=warning  WriteAfterReadMsg=warning  InitialValue=2  ShowAdditionalParam=off
  Data Store Memory2 : DataStoreMemory  DataStoreName=settledTime  ReadBeforeWriteMsg=warning  WriteAfterWriteMsg=warning  WriteAfterReadMsg=warning  ShowAdditionalParam=off  OutDataTypeStr=double  Dimensions=1
  Data Store Read3 : DataStoreRead  DataStoreName=straightDistTraveled
  Data Store Read4 : DataStoreRead  DataStoreName=PID_DIST_TOLERANCE
  Data Store Read5 : DataStoreRead  DataStoreName=PID_SETTLE_TIME
  Data Store Read6 : DataStoreRead  DataStoreName=settledTime
  Data Store Write1 : DataStoreWrite  DataStoreName=leftMotor
  Data Store Write2 : DataStoreWrite  DataStoreName=rightMotor
  Data Store Write3 : DataStoreWrite  DataStoreName=moveDir
  GreaterThanOrEqual1 : RelationalOperator  OutDataTypeStr=boolean  RndMeth=Simplest
  MATLAB Function : MATLAB Function  TreatAsAtomicUnit=on
  PID Controller : pid_lib/PID Controller  Controller=P  Form=Parallel  TimeDomain=Discrete-time  UseExternalTs=on  SampleTime=0.1  IntegratorMethod=Forward Euler  FilterMethod=Forward Euler  ControllerParametersSource=internal  P=100  I=2  D=0.5  UseFilter=on  N=100  TunerSelectOption=Transfer Function Based (PID Tuner App)  InitialConditionSource=internal  InitialConditionForIntegrator=0  InitialConditionForFilter=0  DifferentiatorICPrevScaledInput=0  ExternalReset=none  TrackingMode=off  Kt=1  LimitOutput=on  SatLimitsSource=internal  UpperSaturationLimit=127  LowerSaturationLimit=-127  LinearizeAsGain=off  AntiWindupMode=none  Kb=1  RndMeth=Nearest  POutMin=[]  POutMax=[]  IOutMin=[]  IOutMax=[]  DOutMin=[]  DOutMax=[]  NOutMin=[]  NOutMax=[]  SumOutMin=[]  SumOutMax=[]  SaturationOutMin=[]  SaturationOutMax=[]  PParamMin=[]  PParamMax=[]  IParamMin=[]  IParamMax=[]  DParamMin=[]  DParamMax=[]  NParamMin=[]  NParamMax=[]  KbParamMin=[]  KbParamMax=[]  KtParamMin=[]  KtParamMax=[]  KbOutMin=[]  KbOutMax=[]  KtOutMin=[]  KtOutMax=[]  IntegratorOutMin=[]  IntegratorOutMax=[]  FilterOutMin=[]  FilterOutMax=[]  SumI1OutMin=[]  SumI1OutMax=[]  SumI2OutMin=[]  SumI2OutMax=[]  SumI3OutMin=[]  SumI3OutMax=[]  SumI4OutMin=[]  SumI4OutMax=[]  SumDOutMin=[]  SumDOutMax=[]  DifferentiatorOutMin=[]  DifferentiatorOutMax=[]  FilterDiffOutCoefMin=[]  FilterDiffOutCoefMax=[]  ReciprocalOutMin=[]  ReciprocalOutMax=[]  SumDenOutMin=[]  SumDenOutMax=[]  SumNumOutMin=[]  SumNumOutMax=[]  DivideOutMin=[]  DivideOutMax=[]  UdiffTsProdOutMin=[]  UdiffTsProdOutMax=[]  NTsProdOutMin=[]  NTsProdOutMax=[]  UintegralTsProdOutMin=[]  UintegralTsProdOutMax=[]  UngainTsProdOutMin=[]  UngainTsProdOutMax=[]  IntegratorContinuousStateAttributes=''  IntegratorStateMustResolveToSignalObject=off  IntegratorRTWStateStorageClass=Auto  FilterContinuousStateAttributes=''  FilterStateMustResolveToSignalObject=off  FilterRTWStateStorageClass=Auto  ParallelPVariant=InternalParameters  IdealPVariant=Disabled  IVariant=Disabled  DVariant=Disabled  IntegratorVariant=Disabled  SatVariant=Enabled  AWVariant=Disabled  PCopyVariant=Disabled  TRVariant=Disabled  FdbkBlocksVariant=Forward  IdealPFdbkVariant=Disabled  SatFdbkVariant=Disabled  DerivativeFilterVariant=Disabled  NVariant=Disabled  NCopyVariant=Disabled_SignalSpec  FilterICVariant=Disabled  IntegratorICVariant=Disabled  ExternalResetVariant=Disabled  TRSumVariant=Passthrough  SumFdbkVariant=Disabled  SumVariant=Passthrough_P  TsampFilterVariant=InternalTs  TsampNgainVariant=Passthrough  TsampIntegralVariant=Disabled  ExternalSaturationOutDataTypeStr=Inherit: Same as second input
  Stateflow1 : Stateflow chart  TreatAsAtomicUnit=on
      settings: PortSchema="{\"entries\":[{\"content\":{\"sides\":[{\"content\":{\"connectorIds\":[\"In2\",\"In1\"]},\"type\":\"ConnectorPlacement.EquallySpacedRectSide\",\"uuid\":\"f923337d-3128-4ed8-bb4f-3ea7b5686e2d\"},{\"content\":{\"connectorIds\":[],\"side\":\"RIGHT\"},\"type\":\"ConnectorPlacement.EquallySpacedRectSide\",\"uuid\":\"39dc7172-a5aa-4f5c-b2a4-4c61f2fa72eb\"},{\"content\":{\"connectorIds\":[],\"side\":\"TOP\"},\"type\":\"ConnectorPlacement.EquallySpacedRectSide\",\"uuid\":\"39425eec-6ca1-4a0a-a982-d9b02b3e3e8f\"},{\"content\":{\"connectorIds\":[],\"side\":\"HIDDEN\"},\"type\":\"ConnectorPlacement.EquallySpacedRectSide\",\"uuid\":\"aee45ecb-1b8b-4c38-bfd6-fdbe8fac54d7\"}]},\"type\":\"ConnectorPlacement.EquallySpacedConnector\",\"uuid\":\"e05cbbda-f452-42ce-8e08-9c45c77a95c5\"}],\"packageUris\":[\"http://schema.mathworks.com/mf0/Connector/R2020b\"],\"version\":\"1.0\"}"
  Subtract : Sum  Inputs=+-
  targetDist : ArgIn  DisableCoverage=on  ArgumentName=targetDist
  distHasSettled : ArgOut  DisableCoverage=on  OutDataTypeStr=boolean  ArgumentName=distHasSettled
  wires:
  MATLAB Function/1(sign) -> Data Store Write3/1
  GreaterThanOrEqual1/1 -> distHasSettled/1
  Data Store Read5/1 -> GreaterThanOrEqual1/2
  Data Store Read4/1 -> Stateflow1/1(TOLERANCE)
  Abs1/1 -> Stateflow1/2(error)
  Data Store Read6/1 -> GreaterThanOrEqual1/1
  Subtract/1 -> Abs1/1, PID Controller/1
  targetDist/1 -> Subtract/1
  PID Controller/1 -> MATLAB Function/1(u), Data Store Write2/1, Data Store Write1/1
  Data Store Read3/1 -> Subtract/2

== system AutonomousModel_V1/Simulink Function2 ==
  note: Sample time for this PID controller is
      | not 0.1 seconds, as it is within a subsystem
  note: PID_SETTLE_TIME is measured in n*0.1 seconds,
      | meaning a value of 5 for this would mean a
      | requirement for the PID to turn the robot should
      | settle for 0.5 seconds before stopping
  hasTurnedToAngle : TriggerPort  TriggerType=function-call  IsSimulinkFunction=on  FunctionName=hasTurnedToAngle  FunctionVisibility=scoped  VariantControl=(inherit)
  Abs : Abs
  Constant : Constant  Commented=on  Value=0.1
  Data Store Memory : DataStoreMemory  DataStoreName=PID_ANGLE_TOLERANCE  ReadBeforeWriteMsg=warning  WriteAfterWriteMsg=warning  WriteAfterReadMsg=warning  InitialValue=0.4  ShowAdditionalParam=off
  Data Store Memory1 : DataStoreMemory  DataStoreName=PID_SETTLE_TIME  ReadBeforeWriteMsg=warning  WriteAfterWriteMsg=warning  WriteAfterReadMsg=warning  InitialValue=.5  ShowAdditionalParam=off
  Data Store Memory2 : DataStoreMemory  DataStoreName=settledTime  ReadBeforeWriteMsg=warning  WriteAfterWriteMsg=warning  WriteAfterReadMsg=warning  ShowAdditionalParam=off  OutDataTypeStr=double  Dimensions=1
  Data Store Read : DataStoreRead  DataStoreName=PID_ANGLE_TOLERANCE
  Data Store Read1 : DataStoreRead  DataStoreName=PID_SETTLE_TIME
  Data Store Read2 : DataStoreRead  DataStoreName=settledTime
  Data Store Read7 : DataStoreRead  DataStoreName=signedRobotAngle
  Data Store Write1 : DataStoreWrite  DataStoreName=turnDir
  Data Store Write4 : DataStoreWrite  DataStoreName=leftMotor
  Data Store Write5 : DataStoreWrite  DataStoreName=rightMotor
  Gain : Gain  Gain=-1
  GreaterThanOrEqual : RelationalOperator  OutDataTypeStr=boolean  RndMeth=Simplest
  MATLAB Function : MATLAB Function  TreatAsAtomicUnit=on
  PID Controller1 : pid_lib/PID Controller  Controller=PI  Form=Parallel  TimeDomain=Discrete-time  UseExternalTs=off  SampleTime=-1  IntegratorMethod=Forward Euler  FilterMethod=Forward Euler  ControllerParametersSource=internal  P=0.812779127376154  I=0  D=0  UseFilter=off  N=100  TunerSelectOption=Transfer Function Based (PID Tuner App)  InitialConditionSource=internal  InitialConditionForIntegrator=0.21807542656823095  InitialConditionForFilter=0  DifferentiatorICPrevScaledInput=0  ExternalReset=none  TrackingMode=off  Kt=1  LimitOutput=on  SatLimitsSource=internal  UpperSaturationLimit=127  LowerSaturationLimit=-127  LinearizeAsGain=off  AntiWindupMode=none  Kb=1  RndMeth=Nearest  POutMin=[]  POutMax=[]  IOutMin=[]  IOutMax=[]  DOutMin=[]  DOutMax=[]  NOutMin=[]  NOutMax=[]  SumOutMin=[]  SumOutMax=[]  SaturationOutMin=[]  SaturationOutMax=[]  PParamMin=[]  PParamMax=[]  IParamMin=[]  IParamMax=[]  DParamMin=[]  DParamMax=[]  NParamMin=[]  NParamMax=[]  KbParamMin=[]  KbParamMax=[]  KtParamMin=[]  KtParamMax=[]  KbOutMin=[]  KbOutMax=[]  KtOutMin=[]  KtOutMax=[]  IntegratorOutMin=[]  IntegratorOutMax=[]  FilterOutMin=[]  FilterOutMax=[]  SumI1OutMin=[]  SumI1OutMax=[]  SumI2OutMin=[]  SumI2OutMax=[]  SumI3OutMin=[]  SumI3OutMax=[]  SumI4OutMin=[]  SumI4OutMax=[]  SumDOutMin=[]  SumDOutMax=[]  DifferentiatorOutMin=[]  DifferentiatorOutMax=[]  FilterDiffOutCoefMin=[]  FilterDiffOutCoefMax=[]  ReciprocalOutMin=[]  ReciprocalOutMax=[]  SumDenOutMin=[]  SumDenOutMax=[]  SumNumOutMin=[]  SumNumOutMax=[]  DivideOutMin=[]  DivideOutMax=[]  UdiffTsProdOutMin=[]  UdiffTsProdOutMax=[]  NTsProdOutMin=[]  NTsProdOutMax=[]  UintegralTsProdOutMin=[]  UintegralTsProdOutMax=[]  UngainTsProdOutMin=[]  UngainTsProdOutMax=[]  IntegratorContinuousStateAttributes=''  IntegratorStateMustResolveToSignalObject=off  IntegratorRTWStateStorageClass=Auto  FilterContinuousStateAttributes=''  FilterStateMustResolveToSignalObject=off  FilterRTWStateStorageClass=Auto  ParallelPVariant=InternalParameters  IdealPVariant=Disabled  IVariant=InternalParameters  DVariant=Disabled  IntegratorVariant=Discrete  SatVariant=Enabled  AWVariant=Passthrough  PCopyVariant=Disabled  TRVariant=Disabled  FdbkBlocksVariant=Forward  IdealPFdbkVariant=Disabled  SatFdbkVariant=Disabled  DerivativeFilterVariant=Disabled  NVariant=Disabled  NCopyVariant=Disabled_SignalSpec  FilterICVariant=Disabled  IntegratorICVariant=InternalICs  ExternalResetVariant=Disabled  TRSumVariant=Passthrough  SumFdbkVariant=Disabled  SumVariant=Sum_PI  TsampFilterVariant=InternalTs  TsampNgainVariant=Passthrough  TsampIntegralVariant=Passthrough  ExternalSaturationOutDataTypeStr=Inherit: Same as second input
  Stateflow : Stateflow chart  TreatAsAtomicUnit=on
      settings: PortSchema="{\"entries\":[{\"content\":{\"sides\":[{\"content\":{\"connectorIds\":[\"In2\",\"In1\"]},\"type\":\"ConnectorPlacement.EquallySpacedRectSide\",\"uuid\":\"f923337d-3128-4ed8-bb4f-3ea7b5686e2d\"},{\"content\":{\"connectorIds\":[],\"side\":\"RIGHT\"},\"type\":\"ConnectorPlacement.EquallySpacedRectSide\",\"uuid\":\"39dc7172-a5aa-4f5c-b2a4-4c61f2fa72eb\"},{\"content\":{\"connectorIds\":[],\"side\":\"TOP\"},\"type\":\"ConnectorPlacement.EquallySpacedRectSide\",\"uuid\":\"39425eec-6ca1-4a0a-a982-d9b02b3e3e8f\"},{\"content\":{\"connectorIds\":[],\"side\":\"HIDDEN\"},\"type\":\"ConnectorPlacement.EquallySpacedRectSide\",\"uuid\":\"aee45ecb-1b8b-4c38-bfd6-fdbe8fac54d7\"}]},\"type\":\"ConnectorPlacement.EquallySpacedConnector\",\"uuid\":\"e05cbbda-f452-42ce-8e08-9c45c77a95c5\"}],\"packageUris\":[\"http://schema.mathworks.com/mf0/Connector/R2020b\"],\"version\":\"1.0\"}"
  Subtract1 : Sum  Inputs=+-
  targetAngle : ArgIn  DisableCoverage=on  ArgumentName=targetAngle
  angleHasSettled : ArgOut  DisableCoverage=on  OutDataTypeStr=boolean  ArgumentName=angleHasSettled
  wires:
  Constant/1 -> ?
  GreaterThanOrEqual/1 -> angleHasSettled/1
  Subtract1/1 -> PID Controller1/1, Abs/1
  PID Controller1/1 -> Data Store Write5/1, Gain/1
  targetAngle/1 -> MATLAB Function/1(wantedAngle), Subtract1/1
  Data Store Read2/1 -> GreaterThanOrEqual/1
  MATLAB Function/1(turnDir) -> Data Store Write1/1
  Gain/1 -> Data Store Write4/1
  Data Store Read/1 -> Stateflow/1(TOLERANCE)
  Data Store Read1/1 -> GreaterThanOrEqual/2
  Abs/1 -> Stateflow/2(error)
  Data Store Read7/1 -> Subtract1/2

== system AutonomousModel_V1/Simulink Function3 ==
  hasMovedToCoords : TriggerPort  TriggerType=function-call  IsSimulinkFunction=on  FunctionName=hasMovedToCoords  FunctionVisibility=scoped  VariantControl=(inherit)
  Stateflow1 : Stateflow chart  AncestorBlock=RoboticsPlayground/Utilities and Hardware/Stateflow  TreatAsAtomicUnit=on
  xCoord : ArgIn  DisableCoverage=on  ArgumentName=xCoord
  yCoord : ArgIn  Port=2  ArgumentName=yCoord
  arrived : ArgOut  DisableCoverage=on  OutDataTypeStr=boolean  ArgumentName=arrived
  wires:
  xCoord/1 -> Stateflow1/1(yCoord)
  Stateflow1/1(hasDrivenToTarget) -> arrived/1
  yCoord/1 -> Stateflow1/2(xCoord)

== system AutonomousModel_V1/Simulink Function4 ==
  dropVaccine : TriggerPort  TriggerType=function-call  IsSimulinkFunction=on  FunctionName=dropVaccine  FunctionVisibility=scoped  VariantControl=(inherit)
  Stateflow1 : Stateflow chart  TreatAsAtomicUnit=on

== system AutonomousModel_V1/Stateflow/getPostChange ==
  robotAngle : Inport  OutDataTypeStr=double  PortDimensions=1
  changeInDist : Inport  Port=2  OutDataTypeStr=double  PortDimensions=1
  xAxisDir : Inport  Port=3  OutDataTypeStr=int8  PortDimensions=1
  yAxisDir : Inport  Port=4  OutDataTypeStr=int8  PortDimensions=1
  f : TriggerPort  TriggerType=function-call  VariantControl=(inherit)
      settings: CopyFcn=Stateflow.SLINSF.SimulinkMan.removeBlockPreDeleteFcn  PreDeleteFcn=Stateflow.SLINSF.SimulinkMan.unsafePredeleteFcn
  Cos : Trigonometry  Operator=cos  OutputSignalType=real
  Degrees to Radians : simulink_extras/Transformations/Degrees to Radians
  Product{,1..3} (4 alike) : Product  RndMeth=Zero
  Sin : Trigonometry  OutputSignalType=real
  deltaX : Outport
  deltaY : Outport  Port=2
  wires:
  robotAngle/1 -> Degrees to Radians/1
  Degrees to Radians/1 -> Cos/1, Sin/1
  changeInDist/1 -> Product1/1, Product/2
  Sin/1 -> Product1/2
  Cos/1 -> Product/1
  xAxisDir/1 -> Product2/1
  Product/1 -> Product2/2
  Product1/1 -> Product3/1
  yAxisDir/1 -> Product3/2
  Product2/1 -> deltaX/1
  Product3/1 -> deltaY/1

== system AutonomousModel_V1/Stateflow1/CALCULATE_DIST.getDistChange ==
  note: 0.5 * TICKS_TO_DIST, where TICKS_TO_DIST = (2*pi*0.1) / 180
  leftTicks : Inport  OutDataTypeStr=double  PortDimensions=1
  rightTicks : Inport  Port=2  OutDataTypeStr=double  PortDimensions=1
  moveDir : Inport  Port=3  OutDataTypeStr=double  PortDimensions=1
  getDistChange : TriggerPort  TriggerType=function-call  VariantControl=(inherit)
      settings: CopyFcn=Stateflow.SLINSF.SimulinkMan.removeBlockPreDeleteFcn  PreDeleteFcn=Stateflow.SLINSF.SimulinkMan.unsafePredeleteFcn
  Add : Sum
  Data Store Read1 : DataStoreRead  DataStoreName=prevLMticks
  Data Store Read7 : DataStoreRead  DataStoreName=prevRMticks
  Multiply : Gain  Gain=0.00174532925  OutDataTypeStr=double  ParamDataTypeStr=Inherit: Same as input
  Product : Product  OutDataTypeStr=double  RndMeth=Zero
  Subtract : Sum  Inputs=+-
  Subtract1 : Sum  Inputs=+-
  distChange : Outport  OutDataTypeStr=double
  wires:
  Subtract/1 -> Add/1
  Data Store Read1/1 -> Subtract/2
  leftTicks/1 -> Subtract/1
  Add/1 -> Product/2
  Product/1 -> distChange/1
  Data Store Read7/1 -> Subtract1/2
  moveDir/1 -> Multiply/1
  Subtract1/1 -> Add/2
  rightTicks/1 -> Subtract1/1
  Multiply/1 -> Product/1

== system AutonomousModel_V1/Stateflow3/MAIN_PROGRAM.PHASE_1.hasClearedPlatformAt ==
  gridX : Inport  OutDataTypeStr=double  PortDimensions=1
  gridY : Inport  Port=2  OutDataTypeStr=double  PortDimensions=1
  f : TriggerPort  TriggerType=function-call  VariantControl=(inherit)
      settings: CopyFcn=Stateflow.SLINSF.SimulinkMan.removeBlockPreDeleteFcn  PreDeleteFcn=Stateflow.SLINSF.SimulinkMan.unsafePredeleteFcn
  platformCleared : Outport

== system AutonomousModel_V1/Stateflow3/MAIN_PROGRAM.PHASE_1.hasDroppedVacAt ==
  xCoord : Inport  OutDataTypeStr=double  PortDimensions=1
  yCoord : Inport  Port=2  OutDataTypeStr=double  PortDimensions=1
  f : TriggerPort  TriggerType=function-call  VariantControl=(inherit)
      settings: CopyFcn=Stateflow.SLINSF.SimulinkMan.removeBlockPreDeleteFcn  PreDeleteFcn=Stateflow.SLINSF.SimulinkMan.unsafePredeleteFcn
  Stateflow : Stateflow chart  TreatAsAtomicUnit=on
  deliveredVac : Outport
  wires:
  xCoord/1 -> Stateflow/1(xCoord)
  yCoord/1 -> Stateflow/2(yCoord)
  Stateflow/1(vaccineDropped) -> deliveredVac/1

== system AutonomousModel_V1/Stateflow3/hasMovedToCoords ==
  xCoord : Inport  OutDataTypeStr=double  PortDimensions=1
  yCoord : Inport  Port=2  OutDataTypeStr=double  PortDimensions=1
  f : TriggerPort  TriggerType=function-call  VariantControl=(inherit)
      settings: CopyFcn=Stateflow.SLINSF.SimulinkMan.removeBlockPreDeleteFcn  PreDeleteFcn=Stateflow.SLINSF.SimulinkMan.unsafePredeleteFcn
  Stateflow : Stateflow chart  AncestorBlock=RoboticsPlayground/Utilities and Hardware/Stateflow  TreatAsAtomicUnit=on
  arrived : Outport
  wires:
  xCoord/1 -> Stateflow/1(yCoord)
  yCoord/1 -> Stateflow/2(xCoord)
  Stateflow/1(hasDrivenToTarget) -> arrived/1

== system AutonomousModel_V1/BEST Robotics 2020 Game (Double-Click)/Arena ==
  Floor : Subsystem
  Lamps : Subsystem
  Mechanism Configuration : sm_lib/Utilities/Mechanism Configuration  UniformGravity=Constant  GravityVector=[0 0 -9.80665]  GravityVectorUnits=m/s^2  GravityUnits=m/s^2  LinearizationDelta=0.001  JointModeTransitionNonlinearIterations=2
  Simscape Bus : SimscapeBus  HierarchyStrings=WallSurface;FloorSurface;Ref
  Solver Configuration : nesl_utility/Solver Configuration  PhysicalDomain=network_engine_domain  SubClassName=solver  LeftPortType=input  RightPortType=generic  Tones=[]  Harmonics=[]  SimulateNoise=off  Profile=off  UseLocalSampling=off  EnableSwitchedLinearOptims=on  FrequencyDomain=off  UseCCode=off  RelTol=0.001  AbsTol=1e-06  MinStep=1e-09  ToWorkspace=off  RevertToSquareIcSolve=off  NumHomotopyIterations=100  PhasorMode=off  PhasorModeNumHarmonics=1  DoDC=off  ResidualTolerance=1e-08  UseLocalSolver=off  LocalSolverChoice=NE_BACKWARD_EULER_ADVANCER  LocalSolverSampleTime=0.0002  DoFixedCost=off  MaxNonlinIter=10  MaxModeIter=2  ComputeImpulses=off  ImpulseIterations=2  LinearAlgebra=Sparse  EquationFormulation=NE_TIME_EF  DelaysMemoryBudget=1024  AutomaticFiltering=off  FilteringTimeConstant=0.001  PartitionStorageMethod=AS_NEEDED  PartitionMemoryBudget=1024  PartitionMethod=FAST
  World Frame : sm_lib/Frames and Transforms/World Frame
  RP-Bus : PMIOPort  Side=Left
  connections:
  World Frame/RConn1 -- Floor/RConn1 -- Mechanism Configuration/RConn1 -- Simscape Bus/LConn3 -- Lamps/RConn1 -- Solver Configuration/RConn1
  Simscape Bus/RConn1 -- RP-Bus/RConn1
  Simscape Bus/LConn2 -- Floor/LConn1
